simulink model "Tractor_SingleTrack_Simulink"  (R2025b)
settings: Solver=VariableStepAuto  StartTime=0.0  StopTime=10.0  RelTol=1e-3
undefined symbols (not defined in the file or in its folder): params, TruckParams
settings Model: Creator=jakub  LastModifiedBy=hielke
settings SolverCC: AlgebraicLoopSolver=TrustRegion
settings DebuggingCC: UnconnectedInputMsg=warning  UnconnectedOutputMsg=warning  UnconnectedLineMsg=warning
settings ModelReferenceCC: EnableRefExpFcnMdlSchedulingChecks=on
settings RTWCC: GPUComputeCapability=3.5

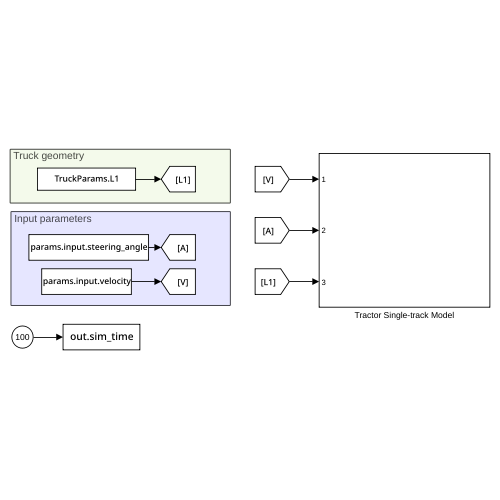
[thumbnail: Simulink's stored preview of the top-level diagram]
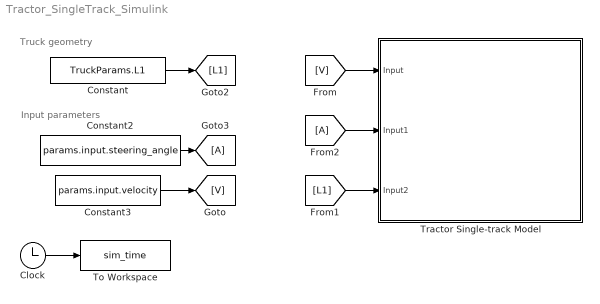
== system Tractor_SingleTrack_Simulink ==
  note: Truck geometry
  note: Input parameters
  Clock : Clock
  Constant : Constant  Value=TruckParams.L1
  Constant2 : Constant  Value=params.input.steering_angle
  Constant3 : Constant  Value=params.input.velocity
  From2 : From
  Goto3 : Goto
  To Workspace : ToWorkspace  VariableName=sim_time  SaveFormat=Timeseries  SampleTime=-1
  Tractor Single-track Model : Subsystem
  wires:
  Clock/1 -> To Workspace/1
  Constant/1 -> [L1]
  Constant2/1 -> Goto3/1
  Constant3/1 -> [V]
  [V] -> Tractor Single-track Model/1(Input)
  [L1] -> Tractor Single-track Model/3(Input2)
  From2/1 -> Tractor Single-track Model/2(Input1)

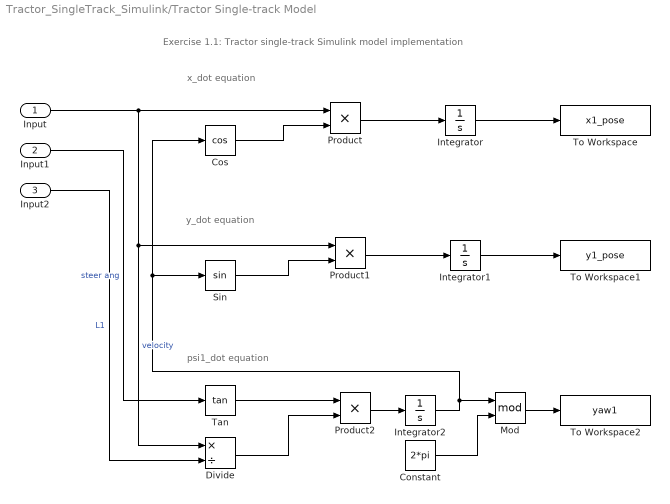
== system Tractor_SingleTrack_Simulink/Tractor Single-track Model ==
  note: Exercise 1.1: Tractor single-track Simulink model implementation
  note: y_dot equation
  note: x_dot equation
  note: psi1_dot equation
  Input : Inport
  Input1 : Inport  Port=2
  Input2 : Inport  Port=3
  Constant : Constant  Value=2*pi
  Cos : Trigonometry  Operator=cos
  Divide : Product  Inputs=*/
  Integrator : Integrator
  Integrator1 : Integrator
  Integrator2 : Integrator
  Mod : Math  Operator=mod
  Product : Product
  Product1 : Product
  Product2 : Product
  Sin : Trigonometry
  Tan : Trigonometry  Operator=tan
  To Workspace : ToWorkspace  VariableName=x1_pose  SaveFormat=Timeseries  SampleTime=-1
  To Workspace1 : ToWorkspace  VariableName=y1_pose  SaveFormat=Timeseries  SampleTime=-1
  To Workspace2 : ToWorkspace  VariableName=yaw1  SaveFormat=Timeseries  SampleTime=-1
  wires:
  Input/1 -> Product/1, Divide/1, Product1/1  "velocity"
  Integrator/1 -> To Workspace/1
  Product/1 -> Integrator/1
  Cos/1 -> Product/2
  Integrator1/1 -> To Workspace1/1
  Product1/1 -> Integrator1/1
  Sin/1 -> Product1/2
  Integrator2/1 -> Mod/1, Cos/1, Sin/1
  Product2/1 -> Integrator2/1
  Input1/1 -> Tan/1  "steer ang"
  Tan/1 -> Product2/1
  Divide/1 -> Product2/2
  Input2/1 -> Divide/2  "L1"
  Constant/1 -> Mod/2
  Mod/1 -> To Workspace2/1
